simulink model "thermostat"  (R2014b)
settings: Solver=FixedStepDiscrete  StartTime=0.0  StopTime=1  FixedStep=0.01  MaxStep=0.0001  RelTol=1e-3
settings Model: Creator=sand080  LastModifiedBy=sand080
settings DataIOCC: LimitDataPoints=off

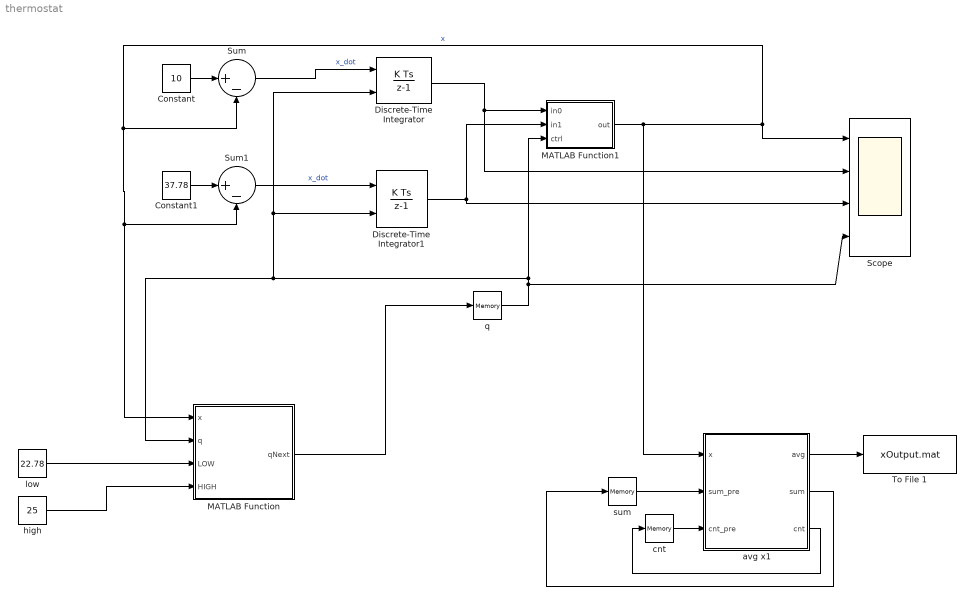
== system thermostat ==
  Constant : Constant  Value=10
  Constant1 : Constant  Value=37.78
  Discrete-Time Integrator : DiscreteIntegrator  ExternalReset=either  InitialCondition=25  InitialConditionSetting=State (most efficient)  SampleTime=-1
  Discrete-Time Integrator1 : DiscreteIntegrator  ExternalReset=either  InitialCondition=22.78  InitialConditionSetting=State (most efficient)  SampleTime=-1
  MATLAB Function : MATLAB Function  TreatAsAtomicUnit=on
  MATLAB Function1 : MATLAB Function  TreatAsAtomicUnit=on
  Scope : Scope  NumInputPorts=4
      settings: TickLabels=on  ShowLegends=on  YMin=22.5~20.5~22.5~-0.5  YMax=25.5~23~25.5~1.5
  Sum : Sum  Inputs=|+-
  Sum1 : Sum  Inputs=|+-
  To File 1 : ToFile  Filename=xOutput.mat
      settings: Decimation=10000000
  avg x1 : MATLAB Function  TreatAsAtomicUnit=on
  cnt : Memory
  high : Constant  Value=25
  low : Constant  Value=22.78
  q : Memory
  sum : Memory
  wires:
  MATLAB Function/1(qNext) -> q/1
  avg x1/2(sum) -> sum/1
  avg x1/3(cnt) -> cnt/1
  cnt/1 -> avg x1/3(cnt_pre)
  sum/1 -> avg x1/2(sum_pre)
  avg x1/1(avg) -> To File 1/1
  Constant/1 -> Sum/1
  Sum/1 -> Discrete-Time Integrator/1  "x_dot"
  Discrete-Time Integrator1/1 -> MATLAB Function1/2(in1), Scope/3
  Constant1/1 -> Sum1/1
  Sum1/1 -> Discrete-Time Integrator1/1  "x_dot"
  Discrete-Time Integrator/1 -> Scope/2, MATLAB Function1/1(in0)
  MATLAB Function1/1(out) -> avg x1/1(x), Scope/1, Sum/2, MATLAB Function/1(x), Sum1/2  "x"
  low/1 -> MATLAB Function/3(LOW)
  high/1 -> MATLAB Function/4(HIGH)
  q/1 -> MATLAB Function1/3(ctrl), Discrete-Time Integrator1/2, Discrete-Time Integrator/2, MATLAB Function/2(q), Scope/4

== matlab function thermostat/MATLAB Function1 ==
  data: in0 input; in1 input; ctrl input; out output
function out = select(in0,in1,ctrl)
%#codegen
if(ctrl==0)
    out=in0;
else
    out=in1;
end

== matlab function thermostat/MATLAB Function ==
  data: x input; q input; qNext output; LOW input; HIGH input
function qNext = phi(x,q, LOW, HIGH)
%#codegen
if q==0 && x> LOW
    qNext=0;
elseif q==0 && x <= LOW
    qNext=1;
elseif q==1 && x < HIGH
    qNext=1;
elseif q==1 && x >= HIGH
    qNext=0;
else
    qNext=2; %this should never execute
end

== matlab function thermostat/avg x1 ==
  data: x input; avg output; sum output; cnt output; sum_pre input; cnt_pre input
function [avg, sum,cnt] = fcn(x,  sum_pre, cnt_pre)
%#codegen

cnt=cnt_pre+1;
sum=sum_pre+x;
avg=sum/cnt;
